simulink model "test_lookup"  (R2020b)
settings: Solver=VariableStepAuto  StartTime=0.0  StopTime=1000.0  RelTol=1e-3
settings Model: Creator=Dogukan  LastModifiedBy=C:\Users\Dogukan

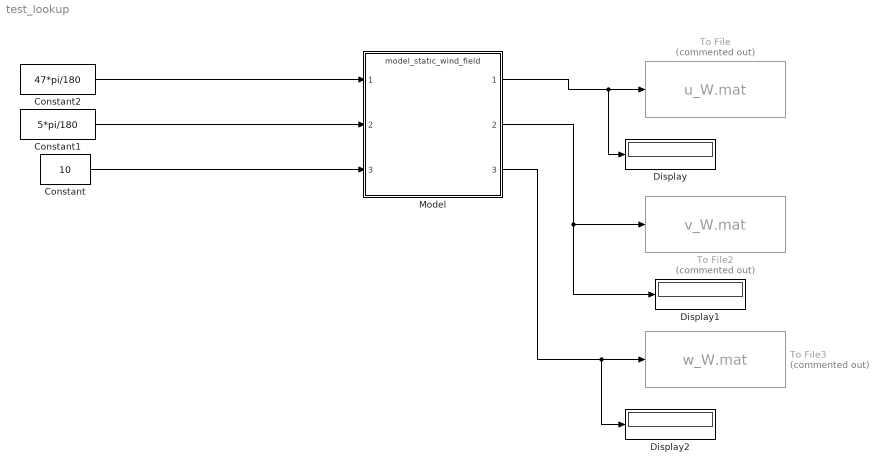
== system test_lookup ==
  Constant : Constant  Value=10  OutDataTypeStr=double
  Constant1 : Constant  Value=5*pi/180
  Constant2 : Constant  Value=47*pi/180
  Display : Display
  Display1 : Display
  Display2 : Display
  Model : ModelReference  ModelNameDialog=model_static_wind_field.slx  SimulationMode=Normal  ModelReferenceVersion=1.29
  To File : ToFile  Commented=on  Filename=u_W.mat  MatrixName=u_W  SaveFormat=Timeseries
  To File2 : ToFile  Commented=on  Filename=v_W.mat  MatrixName=v_W  SaveFormat=Timeseries
  To File3 : ToFile  Commented=on  Filename=w_W.mat  MatrixName=w_W  SaveFormat=Timeseries
  wires:
  Constant/1 -> Model/3
  Constant1/1 -> Model/2
  Constant2/1 -> Model/1
  Model/1 -> Display/1, To File/1
  Model/2 -> To File2/1, Display1/1
  Model/3 -> Display2/1, To File3/1
